simulink model "sim_friction_model"  (R2015b)
settings: Solver=VariableStepAuto  StartTime=0.0  StopTime=10  FixedStep=0.001  RelTol=1e-3
undefined symbols (not defined in the file): lin_sys_A, lin_sys_B, lin_sys_C, lin_sys_D, lin_sys_X
(part 2 of 2)

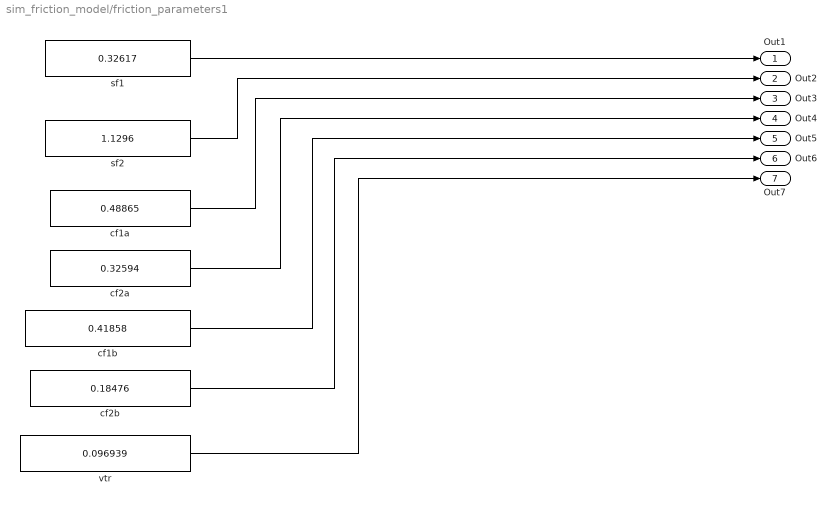
== system sim_friction_model/friction_parameters1 ==
  cf1a : Constant  Value=0.48865
  cf1b : Constant  Value=0.41858
  cf2a : Constant  Value=0.32594
  cf2b : Constant  Value=0.18476
  sf1 : Constant  Value=0.32617
  sf2 : Constant  Value=1.1296
  vtr : Constant  Value=0.096939
  Out1 : Outport
  Out2 : Outport  Port=2
  Out3 : Outport  Port=3
  Out4 : Outport  Port=4
  Out5 : Outport  Port=5
  Out6 : Outport  Port=6
  Out7 : Outport  Port=7
  wires:
  vtr/1 -> Out7/1
  cf2b/1 -> Out6/1
  cf1b/1 -> Out5/1
  cf2a/1 -> Out4/1
  cf1a/1 -> Out3/1
  sf2/1 -> Out2/1
  sf1/1 -> Out1/1

== matlab function sim_friction_model/Stribeck - Dry friction2 ==
  data: F_e input; F_dry output; v input
function F_dry = fcn(F_e,v)
%#codegen

F_s = 0.4; % stiction
F_c = F_s*0.9; % coloumb friction
F_v = 0; % kinetic


sig_s = 1; % model param
gamma = 0.1; % model param

abs_F_e = abs(F_e);

if(v == 0 && abs_F_e < F_s)
    F_dry = F_e;
elseif(v == 0 && abs_F_e >= F_s)
    F_dry = F_s * sign(F_e);
elseif(v > 0)
    F_dry = F_c + (F_s - F_c) * exp(-gamma * v)^sig_s + F_v * v;
else % v < 0
    F_dry = -F_c + (F_c - F_s) * exp(gamma * v)^sig_s + F_v * v;

%     F_dry = (F_c + (F_s - F_c)*exp((-abs(v)*gamma).^sig_s)) * sign(v);
end

== matlab function sim_friction_model/Simple - Dry friction1 ==
  data: F_e input; F_dry output; v input; Fs1 input; Fs2 input; Fc1 input; Fc2 input; Fc1_low input; Fc2_low input; v_treshold input
function F_dry = fcn(F_e,v, Fs1, Fs2, Fc1, Fc2, Fc1_low, Fc2_low, v_treshold)
%#codegen

dz = 0.001;
v_abs = abs(v);
F_e_abs = abs(F_e);

%%%%%%%%%%%
%Vtr_a = 0.5;
%Vtr_b = 1;
% F_s = 0.8; % 5 [N] / 4.23 [N/V] = [V]  stiction 
% F_c = 0.1; % 1st regime
% F_c = 0.4; %F_s * 0.5; % 0.5
% F_v = 0; % kinetic



%v_treshold = 0.5
% Fc1_low = Fc2_low = 0.4 * Fc1

if(v_abs < v_treshold)
    Fc1 = Fc1 * Fc1_low;
    Fc2 = Fc2 * Fc2_low;
end


if(v > 0) % positive velocity
    if(v_abs <= dz && F_e_abs < Fs1) 
        F_dry = F_e;
    elseif(v_abs <= dz && F_e_abs >= Fs1)
        F_dry = Fs1 * sign(F_e); % Stiction
    else
        F_dry = Fc1; % Positive direction couloumb friction
    end
else % negative velocity
   if(v_abs <= dz && F_e_abs < Fs2) 
        F_dry = F_e;
    elseif(v_abs <= dz && F_e_abs >= Fs2)
        F_dry = Fs2 * sign(F_e); % Stiction
    else
        F_dry = Fc2 * -1; % Negative direction couloumb friction
    end 
end





end

== matlab function sim_friction_model/Stribeck - Dry friction + Deadzone ==
  data: F_e input; F_dry output; v input
function F_dry = fcn(F_e,v)
%#codegen

% F_s = 0.4; % stiction

% recalculate stiction and coloumb friction
F_e_max = 3;
F_e_min = 1;

F_s_max = 0.4;
F_s_min = 0.3;

smernice = (F_s_max - F_s_min)/(F_e_max - F_e_min);

F_e_abs = abs(F_e);

if(F_e_abs < F_e_min)
    F_s = F_s_max;
elseif(F_e_abs >= F_e_min && F_e_abs <= F_e_max)
    F_s = F_s_max - (F_e_abs-1) * smernice;
else % > F_e_max
    F_s = F_s_min;
end
    


F_c = F_s*0.9; % coloumb friction
F_v = 0; % kinetic

sig_s = 1; % model param
gamma = 0.1; % model param

dz = 0.001;
v_abs = abs(v);

if(v_abs <= dz && F_e_abs < F_s)
    F_dry = F_e;
%     F_dry = F_s * sign(F_e);
elseif(v_abs <= dz && F_e_abs >= F_s)
    F_dry = F_s * sign(F_e);
    
else
    F_dry = (F_c + (F_s - F_c) * exp(-gamma * v_abs)^sig_s + F_v * v_abs)*sign(v);
end
